simulink model "s1"  (R2024a)
settings: Solver=VariableStepAuto  StartTime=0.0  StopTime=25  RelTol=1e-3
settings Model: Creator=gm54508  LastModifiedBy=gm54508

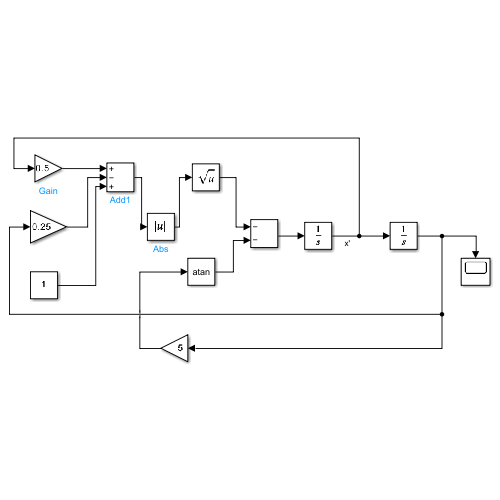
[thumbnail: Simulink's stored preview of the top-level diagram]
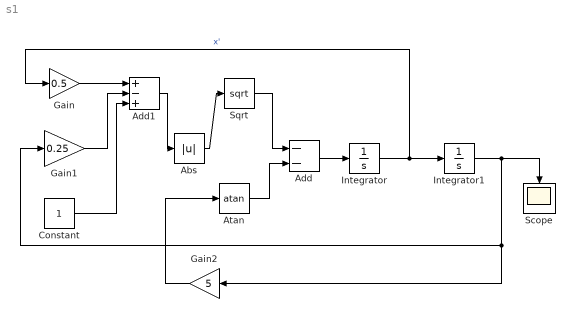
== system s1 ==
  Abs : Abs  SaturateOnIntegerOverflow=off
  Add : Sum  Inputs=--
  Add1 : Sum  Inputs=+-+
  Atan : Trigonometry  Operator=atan
  Constant : Constant
  Gain : Gain  Gain=0.5
  Gain1 : Gain  Gain=0.25
  Gain2 : Gain  Gain=5
  Integrator : Integrator
  Integrator1 : Integrator  InitialCondition=1
  Scope : Scope
  Sqrt : Sqrt
  wires:
  Integrator/1 -> Gain/1, Integrator1/1  "x'"
  Add/1 -> Integrator/1
  Abs/1 -> Sqrt/1
  Gain/1 -> Add1/1
  Gain1/1 -> Add1/2
  Integrator1/1 -> Scope/1, Gain2/1, Gain1/1
  Constant/1 -> Add1/3
  Atan/1 -> Add/2
  Gain2/1 -> Atan/1
  Add1/1 -> Abs/1
  Sqrt/1 -> Add/1
